simulink model "fig10_53and54a"  (Simulink 7.9)
settings: Solver=ode23  SolverMode=SingleTasking  StartTime=0.0  StopTime=20.0  RelTol=1e-3  AbsTol=1e-5
settings Model: Creator=abbas  LastModifiedBy=abbas  ExtModeTrigMode=oneshot  ExtModeArmWhenConnect=off
settings DataIOCC: LimitDataPoints=off
settings OptimizationCC: BlockReduction=off  BooleanDataType=off  InlineInvariantSignals=on  InitFltsAndDblsToZero=on
settings DebuggingCC: SaveWithParameterizedLinksMsg=none  SignalResolutionControl=TryResolveAllWithWarning  SolverPrmCheckMsg=none  MultiTaskDSMMsg=warning  MultiTaskCondExecSysMsg=none  FcnCallInpInsideContextMsg=Use local settings  StrictBusMsg=None
settings HardwareCC: TargetUnknown=on
settings RTWCC: IncludeERTFirstTime=on
settings GRTTargetCC: TargetFcnLib=ansi_tfl_tmw.mat  ModelReferenceCompliant=off  CombineOutputUpdateFcns=off  MatFileLogging=off  GRTInterface=on

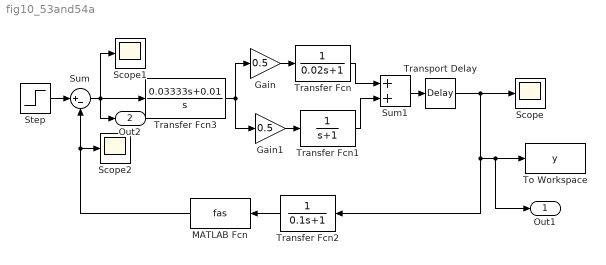
== system fig10_53and54a ==
  Gain : Gain  Gain=0.5  SaturateOnIntegerOverflow=on  OutDataTypeStr=Inherit: Same as input  ParamDataTypeStr=Inherit: Same as input
  Gain1 : Gain  Gain=0.5  SaturateOnIntegerOverflow=on  OutDataTypeStr=Inherit: Same as input  ParamDataTypeStr=Inherit: Same as input
  MATLAB Fcn : MATLABFcn  MATLABFcn=fas  OutputDimensions=1
  Scope : Scope
      settings: TickLabels=on
  Scope1 : Scope
      settings: TickLabels=on
  Scope2 : Scope
      settings: TickLabels=on
  Step : Step  Time=0  After=0.5
  Sum : Sum  Inputs=|+-  SaturateOnIntegerOverflow=on  InputSameDT=on  OutDataTypeStr=Inherit: Same as first input
  Sum1 : Sum  SaturateOnIntegerOverflow=on  InputSameDT=on  OutDataTypeStr=Inherit: Same as first input
  To Workspace : ToWorkspace  VariableName=y  SampleTime=-1
  Transfer Fcn : TransferFcn  Denominator=[0.02 1]
  Transfer Fcn1 : TransferFcn  Denominator=[1 1]
  Transfer Fcn2 : TransferFcn  Denominator=[0.1 1]
  Transfer Fcn3 : TransferFcn  Numerator=[0.03333 0.01]  Denominator=[1 0]
  Transport Delay : TransportDelay  DelayTime=0.2
  Out1 : Outport
  Out2 : Outport  Port=2
  wires:
  Transfer Fcn1/1 -> Sum1/2
  Sum1/1 -> Transport Delay/1
  Transport Delay/1 -> Scope/1, Transfer Fcn2/1, To Workspace/1, Out1/1
  Transfer Fcn/1 -> Sum1/1
  Gain/1 -> Transfer Fcn/1
  Transfer Fcn3/1 -> Gain/1, Gain1/1
  Gain1/1 -> Transfer Fcn1/1
  Transfer Fcn2/1 -> MATLAB Fcn/1
  MATLAB Fcn/1 -> Scope2/1, Sum/2
  Step/1 -> Sum/1
  Sum/1 -> Transfer Fcn3/1, Scope1/1, Out2/1
